simulink model "p7simulink"  (R2025b)
settings: Solver=VariableStepAuto  StartTime=0.0  StopTime=10.0  RelTol=1e-3
settings Model: Creator=raul  LastModifiedBy=raul

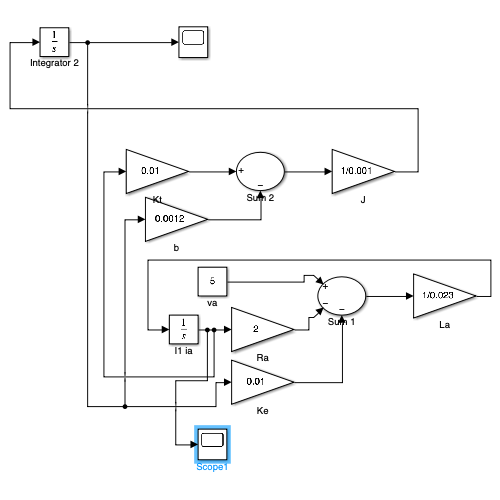
[thumbnail: Simulink's stored preview of the top-level diagram]
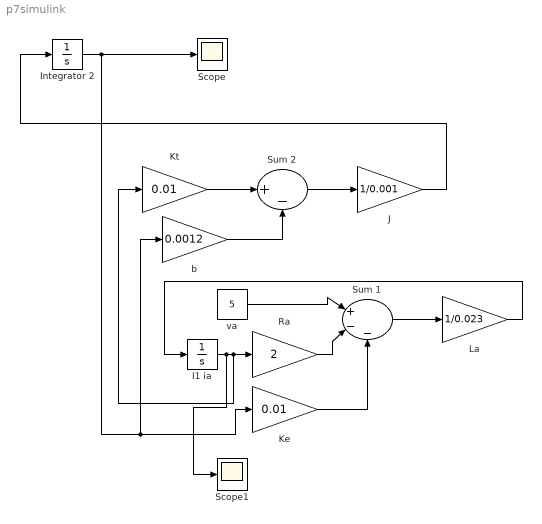
== system p7simulink ==
  I1 ia : Integrator
  Integrator 2 : Integrator
  J : Gain  Gain=1/0.001
  Ke : Gain  Gain=0.01
  Kt : Gain  Gain=0.01
  La : Gain  Gain=1/0.023
  Ra : Gain  Gain=2
  Scope : Scope
      settings: ActiveDisplayYMinimum=-2.5000247365856443  ActiveDisplayYMaximum=22.5002226292708
  Scope1 : Scope
      settings: ActiveDisplayYMinimum=-0.31135315049383205  ActiveDisplayYMaximum=2.8021783544444889
  Sum 1 : Sum  Inputs=|+--
  Sum 2 : Sum  Inputs=|+-
  b : Gain  Gain=0.0012
  va : Constant  Value=5
  wires:
  va/1 -> Sum 1/1
  Ra/1 -> Sum 1/2
  Sum 1/1 -> La/1
  Ke/1 -> Sum 1/3
  Kt/1 -> Sum 2/1
  b/1 -> Sum 2/2
  Integrator 2/1 -> Ke/1, b/1, Scope/1
  Sum 2/1 -> J/1
  J/1 -> Integrator 2/1
  La/1 -> I1 ia/1
  I1 ia/1 -> Scope1/1, Kt/1, Ra/1
